simulink model "lqg"  (R2017a)
settings: Solver=VariableStepAuto  StartTime=0.0  StopTime=30  RelTol=1e-3
values from neighbouring files (symbols this model uses):
  A = [0 0 0 1;0 0 1 0;0 0 0 0;0 0 0 0]    [Sphero_model.m]
  B = [0 0;0 0;1 0;0 1]    [Sphero_model.m]
  C = eye(4)    [Sphero_model.m]
  D = [0 0;0 0;0 0;0 0]    [Sphero_model.m]
undefined symbols (not defined in the file or in its folder): F1, F2, Fi, L, v
settings Model: Creator=Zichong Lu  LastModifiedBy=Zichong Lu

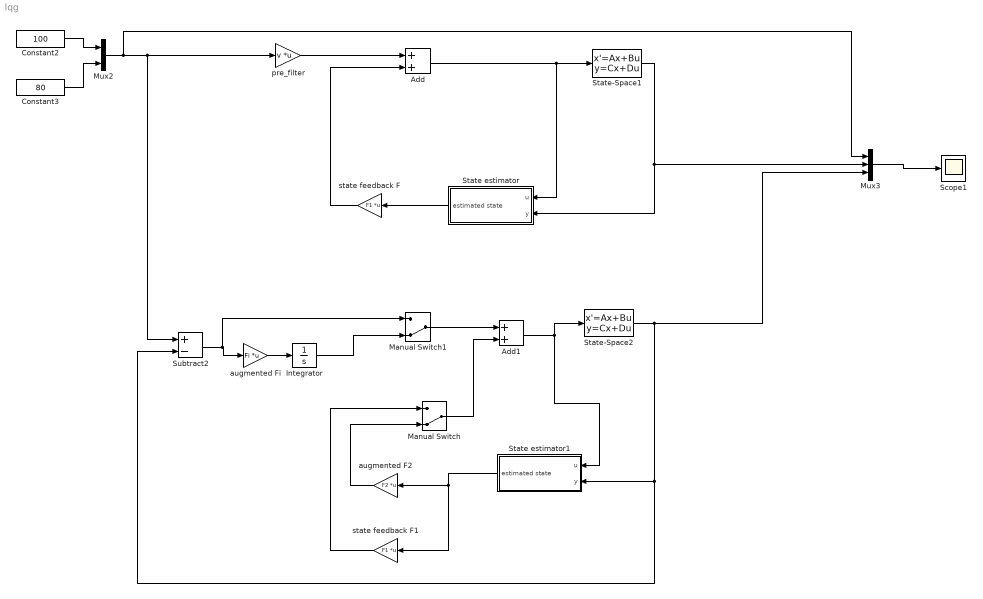
== system lqg ==
  Add : Sum
  Add1 : Sum
  Constant2 : Constant  Value=100
  Constant3 : Constant  Value=80
  Integrator : Integrator
  Manual Switch : ManualSwitch  CurrentSetting=0
  Manual Switch1 : ManualSwitch  CurrentSetting=0
  Mux2 : Mux  Inputs=2
  Mux3 : Mux  Inputs=3
  Scope1 : Scope
  State estimator : Subsystem
  State estimator1 : Subsystem
  State-Space1 : StateSpace  A=A  B=B  C=C  D=C  X0=0
  State-Space2 : StateSpace  A=A  B=B  C=C  D=D  X0=0
  Subtract2 : Sum  Inputs=+-
  augmented F2 : Gain  Gain=F2  Multiplication=Matrix(K*u) (u vector)
  augmented Fi : Gain  Gain=Fi  Multiplication=Matrix(K*u) (u vector)
  pre_filter : Gain  Gain=v  Multiplication=Matrix(K*u) (u vector)
  state feedback F : Gain  Gain=F1  Multiplication=Matrix(K*u) (u vector)
  state feedback F1 : Gain  Gain=F1  Multiplication=Matrix(K*u) (u vector)
  wires:
  Mux3/1 -> Scope1/1
  Constant2/1 -> Mux2/1
  Constant3/1 -> Mux2/2
  Add/1 -> State-Space1/1, State estimator/1(u)
  State estimator/1(estimated state) -> state feedback F/1
  state feedback F/1 -> Add/2
  pre_filter/1 -> Add/1
  Subtract2/1 -> Manual Switch1/1, augmented Fi/1
  state feedback F1/1 -> Manual Switch/1
  State-Space2/1 -> Mux3/3, Subtract2/2, State estimator1/2(y)
  State estimator1/1(estimated state) -> augmented F2/1, state feedback F1/1
  Add1/1 -> State-Space2/1, State estimator1/1(u)
  Integrator/1 -> Manual Switch1/2
  augmented Fi/1 -> Integrator/1
  Manual Switch/1 -> Add1/2
  augmented F2/1 -> Manual Switch/2
  Manual Switch1/1 -> Add1/1
  Mux2/1 -> Mux3/1, Subtract2/1, pre_filter/1
  State-Space1/1 -> Mux3/2, State estimator/2(y)

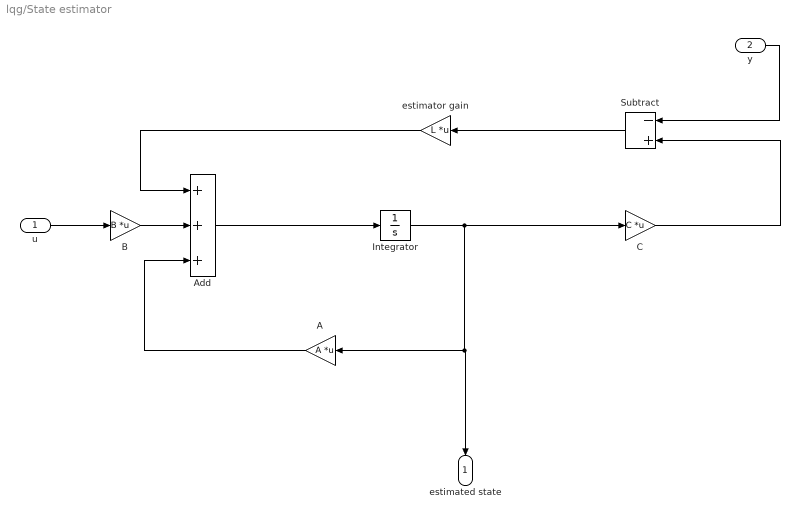
== system lqg/State estimator ==
  u : Inport
  y : Inport  Port=2
  A : Gain  Gain=A  Multiplication=Matrix(K*u) (u vector)
  Add : Sum  Inputs=3
  B : Gain  Gain=B  Multiplication=Matrix(K*u) (u vector)
  C : Gain  Gain=C  Multiplication=Matrix(K*u) (u vector)
  Integrator : Integrator
  Subtract : Sum  Inputs=-+
  estimator gain : Gain  Gain=L  Multiplication=Matrix(K*u) (u vector)
  estimated state : Outport
  wires:
  u/1 -> B/1
  B/1 -> Add/2
  Add/1 -> Integrator/1
  A/1 -> Add/3
  Integrator/1 -> estimated state/1, A/1, C/1
  y/1 -> Subtract/1
  C/1 -> Subtract/2
  Subtract/1 -> estimator gain/1
  estimator gain/1 -> Add/1

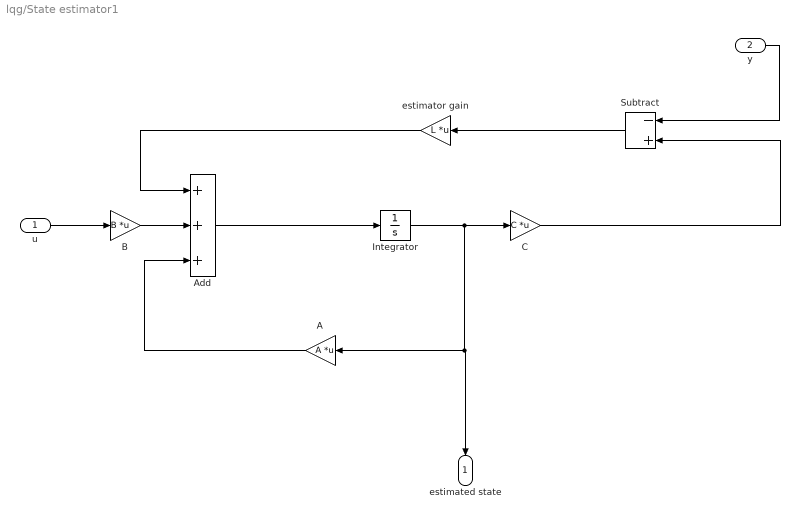
== system lqg/State estimator1 ==
  u : Inport
  y : Inport  Port=2
  A : Gain  Gain=A  Multiplication=Matrix(K*u) (u vector)
  Add : Sum  Inputs=3
  B : Gain  Gain=B  Multiplication=Matrix(K*u) (u vector)
  C : Gain  Gain=C  Multiplication=Matrix(K*u) (u vector)
  Integrator : Integrator
  Subtract : Sum  Inputs=-+
  estimator gain : Gain  Gain=L  Multiplication=Matrix(K*u) (u vector)
  estimated state : Outport
  wires:
  u/1 -> B/1
  B/1 -> Add/2
  Add/1 -> Integrator/1
  A/1 -> Add/3
  Integrator/1 -> estimated state/1, A/1, C/1
  y/1 -> Subtract/1
  Subtract/1 -> estimator gain/1
  estimator gain/1 -> Add/1
  C/1 -> Subtract/2
